simulink model "HumanoidModel_ResidualRL"  (R2025b)
settings: Solver=daessc  StartTime=0.0  StopTime=11  RelTol=1e-3  AbsTol=1e-3
PreLoadFcn:
  | addpath(fullfile('ImportedURDFSupport','Geometries'));
  | addpath(fullfile('ImportedURDFSupport','Data'));
undefined symbols (not defined in the file): kd_ankle_vy, kd_ankle_wx, kd_hip_sag_vx, kd_hip_sag_wy, kd_hip_vy, kd_hip_vz, kd_hip_wx, kp_ankle_qx, kp_ankle_y, kp_hip_dz, kp_hip_qx, kp_hip_sag_qy, kp_hip_sag_x, kp_hip_y, params, residualRLActionPenaltyWeight, residualRLActionRatePenaltyWeight, residualRLAliveReward, residualRLChannelMap, residualRLEnabled, residualRLLeftFootLoadMap, residualRLManualAction, residualRLNominalFootLoad_N, residualRLObservationInverseScales, residualRLRewardStateWeights, residualRLRightFootLoadMap, residualRLSampleTime_s, residualRLTerminalPenalty, residualRLTorqueLimit_Nm, residualRLUseAgent, robustnessForceDuration_s, robustnessForceStart_s, robustnessForceVector_N, Rx_ref, u_ankle_pitch, u_hip_frontal, u_hip_sagittal, u_knee, u_shoulder_frontal, X, Y, y_ref, Z
libraries: sm_lib x155, nesl_utility x96, simulink_extras x18, simulink x5, robotmaniplib x1, rllib x1
(part 1 of 6)
CloseFcn:
  | rmpath(fullfile('ImportedURDFSupport','Geometries'));
  | rmpath(fullfile('ImportedURDFSupport','Data'));
  | clear simlogImportedURDF
settings Model: Creator=The MathWorks, Inc.  LastModifiedBy=EE_LAPTOP_1137
settings SolverCC: AllowMultiTaskInputOutput=on  AlgebraicLoopSolver=TrustRegion
settings OptimizationCC: EnhancedBackFolding=on  OptimizeBlockOrder=speed  DifferentSizesBufferReuse=on  OptimizationCustomize=off
settings DebuggingCC: UnconnectedInputMsg=warning  UnconnectedOutputMsg=warning  UnconnectedLineMsg=warning  SubsystemReferenceDiagnosticForUnitTest=warning  ArithmeticOperatorsInVariantConditions=warning
settings ModelReferenceCC: EnableRefExpFcnMdlSchedulingChecks=on
settings SFSimCC: SimUseLocalCustomCode=off  CustomCodeUndefinedFunction=UseInterfaceOnly
settings RTWCC: RTWUseLocalCustomCode=off  GPUComputeCapability=3.5  DLArmComputeVersion=19.05
settings SimscapeCC: SimscapeLogType=all  SimscapeLogSimulationStatistics=on  SimscapeLogName=simlogImportedURDF  SimscapeLogLimitData=off  SimscapeLogDataHistory=10000.0
settings ExplorerConfigSet: InternalSimMechanicsExplorerSettings="<ExplorerConfiguration><canonicalview>default</canonicalview><AnimationSetting><BasePlaybackSpeed>1.0</BasePlaybackSpeed><PlaybackSpeedFactor>1.0</PlaybackSpeedFactor></AnimationSetting><TilePanel><TileInfo><Tiles Columns=\"1\" Count=\"1\" Rows=\"1\"><Column Weight=\"1\"/><Row Weight=\"1\"/><Tile Height=\"1\" Width=\"1\" X=\"0\" Y=\"0\"/></Tiles></TileInfo><SceneInfo><SceneViewer><BGColor><R>0.60000002384185791</R><G>0.60000002384185791</G><B>0.60000002384185791</B></BGColor><Camera><DoPerspective>off</DoPerspective><Position><X>0.568799300004328878</X><Y>-0.586338342699650017</Y><Z>0.364238790575057481</Z></Position><Center><X>-0.00855096918529698463</X><Y>-0.00898807351002428589</Y><Z>-0.213111478614568334</Z></Center><Up><X>-0.408248290463863073</X><Y>0.408248290463863073</Y><Z>0.816496580927726145</Z></Up><ViewLimDist>1</ViewLimDist><YLim>0.2580841216444969</YLim><XLim>0.471925251007080049</XLim></Camera></SceneViewer></SceneInfo></TilePanel><MechEditorPanel><Cameras/><GfxPanelCameraMap/><VideoCreator><PlaybackSpeedRatio>1.0</PlaybackSpeedRatio><FrameRate>30</FrameRate><VideoFormat>Motion JPEG AVI</VideoFormat><FrameSize>auto</FrameSize></VideoCreator></MechEditorPanel></ExplorerConfiguration>"

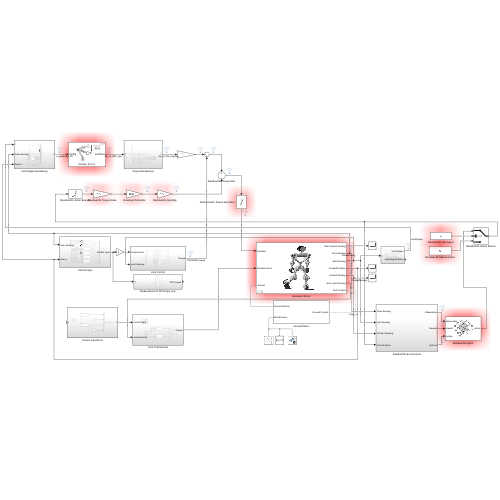
[thumbnail: Simulink's stored preview of the top-level diagram]
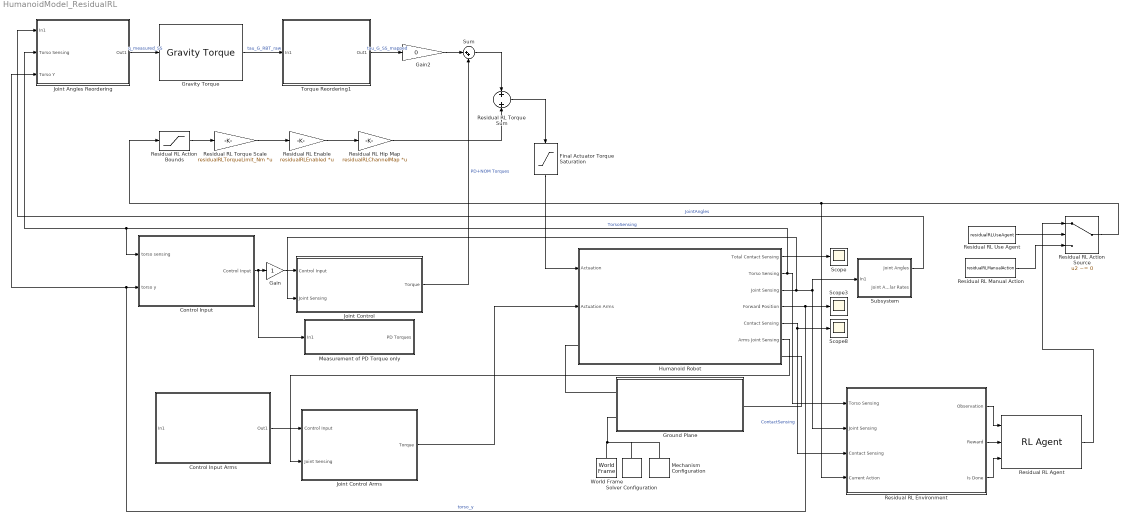
== system HumanoidModel_ResidualRL ==
  Control Input : Subsystem
  Control Input Arms : Subsystem
  Final Actuator Torque Saturation : Saturate  UpperLimit=params.torqueLimits.legActuator  LowerLimit=-params.torqueLimits.legActuator
  Gain : Gain
  Gain2 : Gain  Gain=0
  Gravity Torque : robotmaniplib/Gravity Torque  RigidBodyTree=robotFull  SimulateUsing=Interpreted execution
  Ground Plane : Subsystem
  Humanoid Robot : Subsystem  AncestorBlock=sm_humanoid_walker_lib/Humanoid Robot  mask{contactRadius=params.contact.contactRadius, contactStiffness=params.contact.stiffness, contactDamping=params.contact.damping, contactTWidth=params.contact.transitionWidth, contactStaticFriction=params.contact.staticFriction, contactDynamicFriction=params.contact.dynamicFriction, contactCriticalVelocity=params.contact.criticalVelocity, footDensity=params.materialProperties.lowerBodyDensity, lowerLegDensity=params.materialProperties.lowerBodyDensity, upperLegDensity=params.materialProperties.lowerBodyDensity, hipDensity=params.materialProperties.lowerBodyDensity, trunkDensity=params.materialProperties.upperBodyDensity, shoulderDensity=params.materialProperties.upperBodyDensity, upperArmDensity=params.materialProperties.upperBodyDensity, lowerArmDensity=params.materialProperties.upperBodyDensity, handDensity=params.materialProperties.upperBodyDensity, headDensity=params.materialProperties.upperBodyDensity, hipUpperLimit=params.jointLimits.hipFrontalUpperLimit, hipLowerLimit=params.jointLimits.hipFrontalLowerLimit, kneeUpperLimit=params.jointLimits.kneeUpperLimit, kneeLowerLimit=params.jointLimits.kneeLowerLimit, ankleUpperLimit=params.jointLimits.ankleUpperLimit, ankleLowerLimit=params.jointLimits.ankleLowerLimit, shoulderFrontalUpperLimit=params.jointLimits.shoulderFrontalUpperLimit, shoulderFrontalLowerLimit=params.jointLimits.shoulderFrontalLowerLimit, shoulderSagittalUpperLimit=params.jointLimits.shoulderSagittalUpperLimit, shoulderSagittalLowerLimit=params.jointLimits.shoulderSagittalLowerLimit}
      mask prompts: contactRadius "Contact Sphere Radius (m)"; contactStiffness "Contact Stiffness (N/m)"; contactDamping "Contact Damping (Ns/m)"; contactTWidth "Contact Tranisiton Region Width (m)"; contactStaticFriction "Contact Static Friction"; contactDynamicFriction "Contact Dynamic Friction"; contactCriticalVelocity "Contact Critical Velocity (m/s)"; footDensity "Foot Density (kg/m^3)"; lowerLegDensity "Lower Leg Density (kg/m^3)"; upperLegDensity "Upper Leg Density (kg/m^3)"; hipDensity "Hip Density (kg/m^3)"; trunkDensity "Trunk Density (kg/m^3)"; shoulderDensity "Shoulder Density (kg/m^3)"; upperArmDensity "Upper Arm Density (kg/m^3)"; lowerArmDensity "Lower Arm Density (kg/m^3)"; handDensity "Hand Density (kg/m^3)"; headDensity "Neck / Head Density (kg/m^3)"; hipUpperLimit "Hip Frontal Upper Limit (deg)"; hipLowerLimit "Hip Frontal Lower Limit (deg)"; kneeUpperLimit "Knee Upper Limit (deg)"; kneeLowerLimit "Knee Lower Limit (deg)"; ankleUpperLimit "Ankle Upper Limit (deg)"; ankleLowerLimit "Ankle Lower Limit (deg)"; shoulderFrontalUpperLimit "Shoulder Frontal Upper Limit (deg)"; shoulderFrontalLowerLimit "Shoulder Frontal Lower Limit (deg)"; shoulderSagittalUpperLimit "Shoulder Sagittal Upper Limit (deg)"; shoulderSagittalLowerLimit "Shoulder Sagittal Lower Limit (deg)"
      mask DialogControl Container4 Prompt: Contact Parameters
      mask DialogControl Container9 Prompt: Material Properties
      mask DialogControl Container12 Prompt: Joint Parameters
      mask Display: image('sm_humanoid_robot.PNG'); % Use "Edit Image" on toolstrip to change.
  Joint Angles Reordering : Subsystem
  Joint Control : Subsystem
  Joint Control Arms : Subsystem
  Measurement of PD Torque only : Subsystem
  Mechanism Configuration : sm_lib/Utilities/Mechanism Configuration  UniformGravity=Constant  GravityVector=[0 0 -9.80665]  GravityVectorUnits=m/s^2  LinearizationDelta=0.001  JointModeTransitionNonlinearIterations=2
  Residual RL Action Bounds : Saturate  UpperLimit=1  LowerLimit=-1
  Residual RL Action Source : Switch  Criteria=u2 ~= 0  SaturateOnIntegerOverflow=off  InputSameDT=off
  Residual RL Agent : rllib/RL Agent  Agent=agentObj  ExternalActionAsInput=off  ProvideLastAction=off  ProvideCumRwd=off  TreatAsDirectFeedthrough=on  UseStrictObservationDataTypes=off
  Residual RL Enable : Gain  Gain=residualRLEnabled  Multiplication=Matrix(K*u)
  Residual RL Environment : Subsystem
  Residual RL Hip Map : Gain  Gain=residualRLChannelMap  Multiplication=Matrix(K*u)
  Residual RL Manual Action : Constant  Value=residualRLManualAction
  Residual RL Torque Scale : Gain  Gain=residualRLTorqueLimit_Nm  Multiplication=Matrix(K*u)
  Residual RL Torque Sum : Sum
  Residual RL Use Agent : Constant  Value=residualRLUseAgent
  Scope : Scope
      settings: ActiveDisplayYMinimum=-1  ActiveDisplayYMaximum=1
  Scope3 : Scope
      settings: ActiveDisplayYMinimum=-1.5819424686950212  ActiveDisplayYMaximum=0.4729027116406388  DataLoggingVariableName=ScopeData3
  Scope8 : Scope
      settings: ActiveDisplayYMinimum=-1  ActiveDisplayYMaximum=1  DataLoggingVariableName=ScopeData9
  Solver Configuration : nesl_utility/Solver Configuration  PhysicalDomain=network_engine_domain  SubClassName=solver  LeftPortType=input  RightPortType=generic  Tones=[]  Harmonics=[]  SimulateNoise=off  Profile=off  UseLocalSampling=off  EnableSwitchedLinearOptims=on  FrequencyDomain=off  UseCCode=off  RelTol=0.001  AbsTol=1e-06  MinStep=1e-09  ToWorkspace=off  RevertToSquareIcSolve=off  NumHomotopyIterations=100  PhasorMode=off  PhasorModeNumHarmonics=1  ConsistencySolver=NEWTON_FTOL  IndexReductionMethod=DerivativeReplacement  DoDC=off  ResidualTolerance=1e-09  ConsistencyTolSource=GLOBAL  ConsistencyAbsTol=0.001  ConsistencyRelTol=0.001  ConsistencyTolFactor=0.001  UseLocalSolver=off  LocalSolverChoice=NE_BACKWARD_EULER_ADVANCER  ResolveIndetEquations=on  FunctionEvalNumThread=1  LocalSolverSampleTime=0.001  DoFixedCost=off  MaxNonlinIter=3  MaxModeIter=2  ComputeImpulses=off  ImpulseIterations=2  LinearAlgebra=auto  LinearAlgebraNumThread=0  EquationFormulation=NE_TIME_EF  DelaysMemoryBudget=1024  AutomaticFiltering=on  FilteringTimeConstant=0.001  PartitionStorageMethod=AS_NEEDED  PartitionMemoryBudget=1024  PartitionMethod=ROBUST  MultibodyUseLocalSolver=off  MultibodyLocalSolverChoice=ODE1  MultibodyLocalSolverSampleTime=0.001
  Subsystem : Subsystem
  Sum : Sum  Inputs=|++
  Torque Reordering1 : Subsystem
  World Frame : sm_lib/Frames and Transforms/World Frame
  wires:
  Humanoid Robot/1(Total Contact Sensing) -> Scope/1
  Humanoid Robot/4(Forward Position) -> Joint Angles Reordering/3(Torso Y), Control Input/2(torso y), Scope3/1  "torso_y"
  Humanoid Robot/2(Torso Sensing) -> Joint Angles Reordering/2(Torso Sensing), Control Input/1(torso sensing), Residual RL Environment/1(Torso Sensing)  "TorsoSensing"
  Humanoid Robot/3(Joint Sensing) -> Residual RL Environment/2(Joint Sensing), Subsystem/1(In1), Joint Control/2(Joint Sensing)
  Control Input/1(Control Input) -> Measurement of PD Torque only/1(In1), Gain/1
  Subsystem/1(Joint Angles) -> Joint Angles Reordering/1(In1)  "JointAngles"
  Gain/1 -> Joint Control/1(Control Input)
  Joint Control/1(Torque) -> Sum/2  "PD+NOM Torques"
  Humanoid Robot/5(Contact Sensing) -> Scope8/1, Residual RL Environment/3(Contact Sensing)  "ContactSensing"
  Gain2/1 -> Sum/1
  Joint Angles Reordering/1(Out1) -> Gravity Torque/1  "q_measured_SS"
  Gravity Torque/1 -> Torque Reordering1/1(In1)  "tau_G_RBT_raw"
  Torque Reordering1/1(Out1) -> Gain2/1  "tau_G_SS_mapped"
  Joint Control Arms/1(Torque) -> Humanoid Robot/2(Actuation Arms)
  Control Input Arms/1(Out1) -> Joint Control Arms/1(Control Input)
  Humanoid Robot/6(Arms Joint Sensing) -> Joint Control Arms/2(Joint Sensing)
  Final Actuator Torque Saturation/1 -> Humanoid Robot/1(Actuation)
  Residual RL Action Bounds/1 -> Residual RL Torque Scale/1
  Residual RL Torque Scale/1 -> Residual RL Enable/1
  Residual RL Enable/1 -> Residual RL Hip Map/1
  Sum/1 -> Residual RL Torque Sum/1
  Residual RL Hip Map/1 -> Residual RL Torque Sum/2
  Residual RL Torque Sum/1 -> Final Actuator Torque Saturation/1
  Residual RL Agent/1 -> Residual RL Action Source/1
  Residual RL Use Agent/1 -> Residual RL Action Source/2
  Residual RL Manual Action/1 -> Residual RL Action Source/3
  Residual RL Action Source/1 -> Residual RL Action Bounds/1, Residual RL Environment/4(Current Action)
  Residual RL Environment/1(Observation) -> Residual RL Agent/1
  Residual RL Environment/2(Reward) -> Residual RL Agent/2
  Residual RL Environment/3(Is Done) -> Residual RL Agent/3
  connections:
  Ground Plane/LConn1 -- Humanoid Robot/LConn1
  Ground Plane/LConn2 -- World Frame/RConn1 -- Solver Configuration/RConn1 -- Mechanism Configuration/RConn1
  Humanoid Robot/RConn1 -- Ground Plane/RConn1

== system HumanoidModel_ResidualRL/Control Input ==
  torso sensing : Inport
  torso y : Inport  Port=2
  Bus Selector : BusSelector  OutputSignals=signal1.qx,signal2.wx,signal2.vy,signal2.dz,signal2.vz,signal1.qy,signal2.wy,signal2.x,signal2.vx
  Constant1 : Constant  Value=u_knee
  Constant{5..6,10..11} (4 alike) : Constant  Value=0
  Constant7 : Constant  Value=u_knee
  Left ankle feedback : Subsystem
  Left hip feedback : Subsystem
  Left hip sagittal feedback : Subsystem
  Mux : Mux  Inputs=12
  PD+NOM U : Scope
      settings: ActiveDisplayYMinimum=-15.774140704017688  ActiveDisplayYMaximum=20.952690020044734  DataLoggingVariableName=ScopeData4
  Right ankle feedback : Subsystem
  Right hip feedback : Subsystem
  Right hip sagittal feedback : Subsystem
  Control Input : Outport
  wires:
  Right hip feedback/1(Out1) -> Mux/1  "Right Hip Frontal"
  Mux/1 -> PD+NOM U/1, Control Input/1
  Constant1/1 -> Mux/2  "Right Knee"
  Right ankle feedback/1(Out1) -> Mux/3  "Right Ankle Pitch"
  Right hip sagittal feedback/1(Out1) -> Mux/4  "Right Hip Sagittal"
  Constant5/1 -> Mux/5  "Right Hip Transverse"
  Constant6/1 -> Mux/6  "Right Ankle Roll"
  Constant7/1 -> Mux/8  "Left Knee"
  Left ankle feedback/1(Out1) -> Mux/9  "Left Ankle Pitch"
  Constant11/1 -> Mux/12  "Left Ankle Roll"
  Constant10/1 -> Mux/11  "Left Hip Transverse"
  Left hip sagittal feedback/1(Out1) -> Mux/10  "Left Hip Sagittal"
  torso sensing/1 -> Bus Selector/1
  Bus Selector/1 -> Left hip feedback/1(qx), Left ankle feedback/1(qx), Right ankle feedback/1(qx), Right hip feedback/1(qx)  "<qx>"
  Bus Selector/2 -> Left ankle feedback/2(wx), Left hip feedback/2(wx), Right ankle feedback/2(wx), Right hip feedback/2(wx)  "<wx>"
  Bus Selector/3 -> Right hip feedback/3(vy), Left hip feedback/3(vy), Left ankle feedback/3(vy), Right ankle feedback/3(vy)  "<vy>"
  torso y/1 -> Left hip feedback/4(y), Left ankle feedback/4(y), Right ankle feedback/4(y), Right hip feedback/4(y)
  Left hip feedback/1(Out1) -> Mux/7  "Left Hip Frontal"
  Bus Selector/4 -> Left hip feedback/5(dz), Right hip feedback/5(dz)  "<dz>"
  Bus Selector/5 -> Left hip feedback/6(vz), Right hip feedback/6(vz)  "<vz>"
  Bus Selector/6 -> Left hip sagittal feedback/1(qy), Right hip sagittal feedback/1(qy)  "<qy>"
  Bus Selector/7 -> Left hip sagittal feedback/2(wy), Right hip sagittal feedback/2(wy)  "<wy>"
  Bus Selector/8 -> Left hip sagittal feedback/3(x), Right hip sagittal feedback/3(x)  "<x>"
  Bus Selector/9 -> Left hip sagittal feedback/4(vx), Right hip sagittal feedback/4(vx)  "<vx>"

== system HumanoidModel_ResidualRL/Control Input Arms ==
  In1 : Inport
  Constant1 : Constant  Value=u_shoulder_frontal
  Constant2 : Constant  Value=u_shoulder_frontal
  Constant3 : Constant  Value=0
  Constant5 : Constant  Value=0
  Mux : Mux
  Out1 : Outport
  wires:
  Mux/1 -> Out1/1
  Constant1/1 -> Mux/1  "Right Shoulder Frontal"
  Constant2/1 -> Mux/3  "Left Shoulder Frontal"
  Constant5/1 -> Mux/2  "Right Shoulder Sagittal"
  Constant3/1 -> Mux/4  "Left Shoulder Sagittal"

== system HumanoidModel_ResidualRL/Ground Plane ==
  Ground : sm_lib/Body Elements/Brick Solid  BrickDimensions=[params.display.planeWidth params.display.planeLength params.display.planeHeight]  BrickDimensionsUnits=m  ExportEntireGeometry=on  InertiaType=CalculateFromGeometry  BasedOnType=Density  Density=1000  DensityUnits=kg/m^3  Mass=1  MassUnits=kg  CenterOfMass=[0 0 0]  CenterOfMassUnits=m  MomentsOfInertia=[1 1 1]  MomentsOfInertiaUnits=kg*m^2  ProductsOfInertia=[0 0 0]  ProductsOfInertiaUnits=kg*m^2  GraphicType=FromGeometry  MarkerShape=Sphere  MarkerSize=10  GraphicVisPropType=SimpleVisualProperties  GraphicDiffuseColor=params.display.floorColour  GraphicOpacity=0.3  GraphicSpecularColor=[0.5 0.5 0.5 1.0]  GraphicAmbientColor=[0.15 0.15 0.15 1.0]  GraphicEmissiveColor=[0.0 0.0 0.0 1.0]  GraphicShininess=75  DoExposeReferenceFrame=on  SerializedFrames=<Frames><Frame><Id>Frame1</Id><Value><Name>GS</Name><Origin><Source>GeometricFeature</Source><FeatureName>+z surface</FeatureName></Origin><PrimaryAxis><DefinedDirection>+Z</DefinedDirection><Source>ReferenceFrame</Source><SourceDirection>+Z</SourceDirection><FeatureName></FeatureName></PrimaryAxis><SecondaryAxis><DefinedDirection>+X</DefinedDirection><Source>ReferenceFrame</Source><SourceDirection>+X</SourceDirection><FeatureName></FeatureName></SecondaryAxis></Value></Frame></Frames>
  Rigid Transform : sm_lib/Frames and Transforms/Rigid Transform  RotationMethod=None  FollAlignAxisA=+X  BaseAlignAxisA=+Y  FollAlignAxisB=+Y  BaseAlignAxisB=+Z  RotationStandardAxis=+Z  RotationAngle=0.0  RotationAngleUnits=deg  RotationArbitraryAxis=[0 0 1]  RotationSequenceAxes=FollowerAxes  RotationSequence=XYX  RotationSequenceAngles=[0 0 0]  RotationSequenceAnglesUnits=deg  RotationMatrix=[1 0 0; 0 1 0; 0 0 1]  Quaternion=[1 0 0 0]  TranslationMethod=StandardAxis  TranslationCartesianOffset=[0 0 0]  TranslationCartesianOffsetUnits=m  TranslationStandardAxis=+Y  TranslationStandardOffset=0.5-(params.display.planeLength/2)  TranslationStandardOffsetUnits=m  TranslationROffset=0  TranslationROffsetUnits=m  TranslationThetaOffset=0  TranslationThetaOffsetUnits=deg  TranslationZOffset=0  TranslationZOffsetUnits=m
  Ground Surface : PMIOPort  Side=Left
  Ground Contact : PMIOPort  Port=2  Side=Right
  World Frame : PMIOPort  Port=3  Side=Left
  connections:
  Ground/LConn1 -- Rigid Transform/LConn1
  Ground/LConn2 -- Ground Contact/RConn1
  Ground/RConn1 -- World Frame/RConn1
  Rigid Transform/RConn1 -- Ground Surface/RConn1

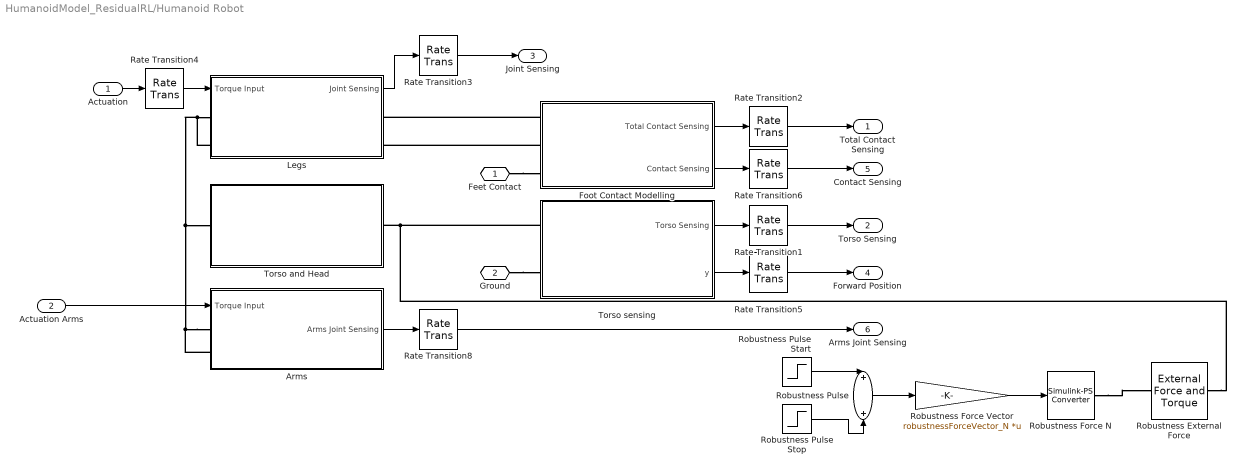
== system HumanoidModel_ResidualRL/Humanoid Robot ==
  Actuation : Inport
  Actuation Arms : Inport  Port=2
  Arms : Subsystem
      mask Display: image('sm_humanoid_arms.PNG'); % Use "Edit Image" on toolstrip to change.
  Foot Contact Modelling : Subsystem
  Legs : Subsystem
      mask Display: image('sm_humanoid_legs.PNG'); % Use "Edit Image" on toolstrip to change.
  Rate Transition{1..6,8} (7 alike) : RateTransition  OutPortSampleTime=params.simulation.Ts
  Robustness External Force : sm_lib/Forces and Torques/External Force and Torque  EnableForceX=off  EnableForceY=off  EnableForceZ=off  EnableForce=on  ForceResolutionFrame=World  EnableTorqueX=off  EnableTorqueY=off  EnableTorqueZ=off  EnableTorque=off  TorqueResolutionFrame=AttachedFrame
  Robustness Force N : nesl_utility/Simulink-PS Converter  PhysicalDomain=network_engine_domain  SubClassName=ps_input  LeftPortType=input  RightPortType=output  PseudoPeriodic=off  Frequencies=[]  NoiseDistribution=none  NoiseParameters=[]  Unit=N  AffineConversion=off  FilteringAndDerivatives=provide  SimscapeFilterOrder=1  InputFilterTimeConstant=0.001  UdotUserProvided=0
  Robustness Force Vector : Gain  Gain=robustnessForceVector_N  Multiplication=Matrix(K*u)
  Robustness Pulse : Sum
  Robustness Pulse Start : Step  Time=robustnessForceStart_s  SampleTime=0
  Robustness Pulse Stop : Step  Time=robustnessForceStart_s + robustnessForceDuration_s  After=-1  SampleTime=0
  Torso and Head : Subsystem
      mask Display: image('sm_humanoid_torso.PNG'); % Use "Edit Image" on toolstrip to change.
  Torso sensing : Subsystem
  Feet Contact : PMIOPort  Side=Right
  " Ground" : PMIOPort  Port=2  Side=Left
  Total Contact Sensing : Outport
  Torso Sensing : Outport  Port=2
  Joint Sensing : Outport  Port=3
  Forward Position : Outport  Port=4
  Contact Sensing : Outport  Port=5
  Arms Joint Sensing : Outport  Port=6
  wires:
  Torso sensing/2(y) -> Rate Transition5/1
  Rate Transition5/1 -> Forward Position/1
  Rate Transition4/1 -> Legs/1(Torque Input)
  Rate Transition3/1 -> Joint Sensing/1
  Rate Transition1/1 -> Torso Sensing/1
  Rate Transition2/1 -> Total Contact Sensing/1
  Torso sensing/1(Torso Sensing) -> Rate Transition1/1
  Actuation/1 -> Rate Transition4/1
  Legs/1(Joint Sensing) -> Rate Transition3/1
  Foot Contact Modelling/1(Total Contact Sensing) -> Rate Transition2/1
  Rate Transition6/1 -> Contact Sensing/1
  Foot Contact Modelling/2(Contact Sensing) -> Rate Transition6/1
  Actuation Arms/1 -> Arms/1(Torque Input)
  Arms/1(Arms Joint Sensing) -> Rate Transition8/1
  Rate Transition8/1 -> Arms Joint Sensing/1
  Robustness Pulse Start/1 -> Robustness Pulse/1
  Robustness Pulse Stop/1 -> Robustness Pulse/2
  Robustness Pulse/1 -> Robustness Force Vector/1
  Robustness Force Vector/1 -> Robustness Force N/1
  connections:
  " Ground"/RConn1 -- Torso sensing/LConn2
  Foot Contact Modelling/LConn2 -- Legs/RConn2
  Foot Contact Modelling/LConn1 -- Legs/RConn1
  Feet Contact/RConn1 -- Foot Contact Modelling/LConn3
  Torso sensing/LConn1 -- Torso and Head/RConn1 -- Robustness External Force/RConn1
  Arms/LConn1 -- Torso and Head/LConn1 -- Legs/LConn1 -- Legs/LConn2 -- Arms/LConn2
  Robustness Force N/RConn1 -- Robustness External Force/LConn1

== system HumanoidModel_ResidualRL/Joint Angles Reordering ==
  In1 : Inport
  Torso Sensing : Inport  Port=2
  Torso Y : Inport  Port=3
  Bus Creator3 : BusCreator  Inputs=22
  Constant : Constant  Value=0
  Demux : Demux  Outputs=12
  Floating Base Selector : BusSelector  OutputSignals=signal2.x,signal2.dz,signal1.qx,signal1.qy,signal1.qz
  Out1 : Outport
  wires:
  In1/1 -> Demux/1
  Bus Creator3/1 -> Out1/1
  Constant/1 -> Bus Creator3/10, Bus Creator3/9, Bus Creator3/8, Bus Creator3/7
  Demux/1 -> Bus Creator3/12  "right_hip_frontal"
  Demux/2 -> Bus Creator3/18  "left_hip_frontal"
  Demux/3 -> Bus Creator3/11  "right_hip_transverse"
  Demux/4 -> Bus Creator3/17  "left_hip_transverse"
  Demux/5 -> Bus Creator3/13  "right_hip_sagittal"
  Demux/6 -> Bus Creator3/19  "left_hip_sagittal"
  Demux/7 -> Bus Creator3/16  "right_ankle_pitch"
  Demux/8 -> Bus Creator3/22  "left_ankle_pitch"
  Demux/9 -> Bus Creator3/15  "right_ankle_roll"
  Demux/10 -> Bus Creator3/21  "left_ankle_roll"
  Demux/11 -> Bus Creator3/14  "right_knee"
  Demux/12 -> Bus Creator3/20  "left_knee"
  Torso Sensing/1 -> Floating Base Selector/1
  Floating Base Selector/1 -> Bus Creator3/1  "<x>"
  Torso Y/1 -> Bus Creator3/2
  Floating Base Selector/2 -> Bus Creator3/3  "<dz>"
  Floating Base Selector/3 -> Bus Creator3/4  "<qx>"
  Floating Base Selector/4 -> Bus Creator3/5  "<qy>"
  Floating Base Selector/5 -> Bus Creator3/6  "<qz>"

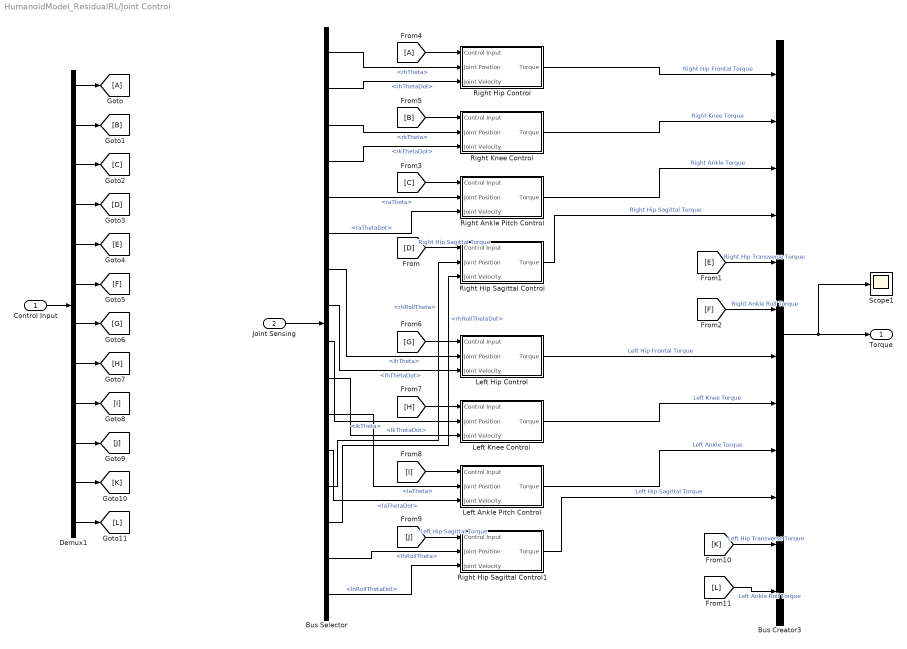
== system HumanoidModel_ResidualRL/Joint Control ==
  Control Input : Inport
  Joint Sensing : Inport  Port=2
  Bus Creator3 : BusCreator  Inputs=12
  Bus Selector : BusSelector  OutputSignals=signal1.signal1.rhTheta,signal1.signal1.rhThetaDot,signal1.signal2.rkTheta,signal1.signal2.rkThetaDot,signal1.signal3.raTheta,signal1.signal3.raThetaDot,signal2.signal1.lhTheta,signal2.signal1.lhThetaDot,signal2.signal2.lkTheta,signal2.signal2.lkThetaDot,signal2.signal3.laTheta,signal2.signal3.laThetaDot,signal1.signal4.rhRollTheta,signal1.signal4.rhRollThetaDot,signal2.signal4.lhRollTheta,signal2.signal4.lhRollThetaDot
  Demux1 : Demux  Outputs=12
  From4 : From
  Goto : Goto
  Left Ankle Pitch Control : Subsystem  AncestorBlock=sm_humanoid_walker_lib/Joint Controller  mask{jointStiffness=params.controller.ankleStiffness, jointDamping=params.controller.ankleDamping, jointUpperLimit=params.jointLimits.ankleUpperLimit, jointLowerLimit=params.jointLimits.ankleLowerLimit, jointTorqueLimit=params.torqueLimits.ankle}
      mask prompts: jointStiffness "Joint Control Stiffness (N*m/rad)"; jointDamping "Joint Control Damping (N*m*s/rad)"; jointUpperLimit "Joint Upper Limit (deg)"; jointLowerLimit "Joint Lower Limt (deg)"; jointTorqueLimit "Joint Absolute Torque Limit (N*m)"
      mask DialogControl DescTextVar Prompt: Stiffness based joint controller.
  Left Hip Control : Subsystem  AncestorBlock=sm_humanoid_walker_lib/Joint Controller  mask{jointStiffness=params.controller.hipFrontalStiffness, jointDamping=params.controller.hipFrontalDamping, jointUpperLimit=params.jointLimits.hipFrontalUpperLimit, jointLowerLimit=params.jointLimits.hipFrontalLowerLimit, jointTorqueLimit=params.torqueLimits.hipFrontal}
      mask prompts: jointStiffness "Joint Control Stiffness (N*m/rad)"; jointDamping "Joint Control Damping (N*m*s/rad)"; jointUpperLimit "Joint Upper Limit (deg)"; jointLowerLimit "Joint Lower Limt (deg)"; jointTorqueLimit "Joint Absolute Torque Limit (N*m)"
      mask DialogControl DescTextVar Prompt: Stiffness based joint controller.
  Left Knee Control : Subsystem  AncestorBlock=sm_humanoid_walker_lib/Joint Controller  mask{jointStiffness=params.controller.kneeStiffness, jointDamping=params.controller.kneeDamping, jointUpperLimit=params.jointLimits.kneeUpperLimit, jointLowerLimit=params.jointLimits.kneeLowerLimit, jointTorqueLimit=params.torqueLimits.knee}
      mask prompts: jointStiffness "Joint Control Stiffness (N*m/rad)"; jointDamping "Joint Control Damping (N*m*s/rad)"; jointUpperLimit "Joint Upper Limit (deg)"; jointLowerLimit "Joint Lower Limt (deg)"; jointTorqueLimit "Joint Absolute Torque Limit (N*m)"
      mask DialogControl DescTextVar Prompt: Stiffness based joint controller.
  Right Ankle Pitch Control : Subsystem  AncestorBlock=sm_humanoid_walker_lib/Joint Controller  mask{jointStiffness=params.controller.ankleStiffness, jointDamping=params.controller.ankleDamping, jointUpperLimit=params.jointLimits.ankleUpperLimit, jointLowerLimit=params.jointLimits.ankleLowerLimit, jointTorqueLimit=params.torqueLimits.ankle}
      mask prompts: jointStiffness "Joint Control Stiffness (N*m/rad)"; jointDamping "Joint Control Damping (N*m*s/rad)"; jointUpperLimit "Joint Upper Limit (deg)"; jointLowerLimit "Joint Lower Limt (deg)"; jointTorqueLimit "Joint Absolute Torque Limit (N*m)"
      mask DialogControl DescTextVar Prompt: Stiffness based joint controller.
  Right Hip Control : Subsystem  AncestorBlock=sm_humanoid_walker_lib/Joint Controller  mask{jointStiffness=params.controller.hipFrontalStiffness, jointDamping=params.controller.hipFrontalDamping, jointUpperLimit=params.jointLimits.hipFrontalUpperLimit, jointLowerLimit=params.jointLimits.hipFrontalLowerLimit, jointTorqueLimit=params.torqueLimits.hipFrontal}
      mask prompts: jointStiffness "Joint Control Stiffness (N*m/rad)"; jointDamping "Joint Control Damping (N*m*s/rad)"; jointUpperLimit "Joint Upper Limit (deg)"; jointLowerLimit "Joint Lower Limt (deg)"; jointTorqueLimit "Joint Absolute Torque Limit (N*m)"
      mask DialogControl DescTextVar Prompt: Stiffness based joint controller.
  Right Hip Sagittal Control : Subsystem  AncestorBlock=sm_humanoid_walker_lib/Joint Controller  mask{jointStiffness=params.controller.hipSagittalStiffness, jointDamping=params.controller.hipSagittalDamping, jointUpperLimit=params.jointLimits.hipSagittalUpperLimit, jointLowerLimit=params.jointLimits.hipSagittalLowerLimit, jointTorqueLimit=params.torqueLimits.hipSagittal}
      mask prompts: jointStiffness "Joint Control Stiffness (N*m/rad)"; jointDamping "Joint Control Damping (N*m*s/rad)"; jointUpperLimit "Joint Upper Limit (deg)"; jointLowerLimit "Joint Lower Limt (deg)"; jointTorqueLimit "Joint Absolute Torque Limit (N*m)"
      mask DialogControl DescTextVar Prompt: Stiffness based joint controller.
  Right Hip Sagittal Control1 : Subsystem  AncestorBlock=sm_humanoid_walker_lib/Joint Controller  mask{jointStiffness=params.controller.hipSagittalStiffness, jointDamping=params.controller.hipSagittalDamping, jointUpperLimit=params.jointLimits.hipSagittalUpperLimit, jointLowerLimit=params.jointLimits.hipSagittalLowerLimit, jointTorqueLimit=params.torqueLimits.hipSagittal}
      mask prompts: jointStiffness "Joint Control Stiffness (N*m/rad)"; jointDamping "Joint Control Damping (N*m*s/rad)"; jointUpperLimit "Joint Upper Limit (deg)"; jointLowerLimit "Joint Lower Limt (deg)"; jointTorqueLimit "Joint Absolute Torque Limit (N*m)"
      mask DialogControl DescTextVar Prompt: Stiffness based joint controller.
  Right Knee Control : Subsystem  AncestorBlock=sm_humanoid_walker_lib/Joint Controller  mask{jointStiffness=params.controller.kneeStiffness, jointDamping=params.controller.kneeDamping, jointUpperLimit=params.jointLimits.kneeUpperLimit, jointLowerLimit=params.jointLimits.kneeLowerLimit, jointTorqueLimit=params.torqueLimits.knee}
      mask prompts: jointStiffness "Joint Control Stiffness (N*m/rad)"; jointDamping "Joint Control Damping (N*m*s/rad)"; jointUpperLimit "Joint Upper Limit (deg)"; jointLowerLimit "Joint Lower Limt (deg)"; jointTorqueLimit "Joint Absolute Torque Limit (N*m)"
      mask DialogControl DescTextVar Prompt: Stiffness based joint controller.
  Scope1 : Scope
      settings: ActiveDisplayYMinimum=-18.809813505018703  ActiveDisplayYMaximum=29.661981385621988  DataLoggingVariableName=ScopeData8
  Torque : Outport
  wires:
  Right Hip Control/1(Torque) -> Bus Creator3/1  "Right Hip Frontal Torque"
  [B] -> Right Knee Control/1(Control Input)
  Bus Creator3/1 -> Scope1/1, Torque/1
  Demux1/3 -> [C]
  [I] -> Left Ankle Pitch Control/1(Control Input)
  Bus Selector/10 -> Left Knee Control/3(Joint Velocity)  "<lkThetaDot>"
  Demux1/1 -> Goto/1
  Right Ankle Pitch Control/1(Torque) -> Bus Creator3/3  "Right Ankle Torque"
  Bus Selector/3 -> Right Knee Control/2(Joint Position)  "<rkTheta>"
  Bus Selector/6 -> Right Ankle Pitch Control/3(Joint Velocity)  "<raThetaDot>"
  Bus Selector/11 -> Left Ankle Pitch Control/2(Joint Position)  "<laTheta>"
  Bus Selector/12 -> Left Ankle Pitch Control/3(Joint Velocity)  "<laThetaDot>"
  [C] -> Right Ankle Pitch Control/1(Control Input)
  Right Knee Control/1(Torque) -> Bus Creator3/2  "Right Knee Torque"
  Bus Selector/4 -> Right Knee Control/3(Joint Velocity)  "<rkThetaDot>"
  Bus Selector/1 -> Right Hip Control/2(Joint Position)  "<rhTheta>"
  [H] -> Left Knee Control/1(Control Input)
  Bus Selector/9 -> Left Knee Control/2(Joint Position)  "<lkTheta>"
  Control Input/1 -> Demux1/1
  Joint Sensing/1 -> Bus Selector/1
  From4/1 -> Right Hip Control/1(Control Input)
  Bus Selector/7 -> Left Hip Control/2(Joint Position)  "<lhTheta>"
  Bus Selector/2 -> Right Hip Control/3(Joint Velocity)  "<rhThetaDot>"
  Demux1/5 -> [E]
  Bus Selector/8 -> Left Hip Control/3(Joint Velocity)  "<lhThetaDot>"
  Demux1/2 -> [B]
  Bus Selector/5 -> Right Ankle Pitch Control/2(Joint Position)  "<raTheta>"
  [G] -> Left Hip Control/1(Control Input)
  Demux1/4 -> [D]
  Demux1/6 -> [F]
  Demux1/7 -> [G]
  Demux1/8 -> [H]
  Demux1/9 -> [I]
  Demux1/10 -> [J]
  Demux1/11 -> [K]
  Demux1/12 -> [L]
  Left Ankle Pitch Control/1(Torque) -> Bus Creator3/9  "Left Ankle Torque"
  Left Knee Control/1(Torque) -> Bus Creator3/8  "Left Knee Torque"
  Left Hip Control/1(Torque) -> Bus Creator3/7  "Left Hip Frontal Torque"
  [L] -> Bus Creator3/12  "Left Ankle Roll Torque"
  [K] -> Bus Creator3/11  "Left Hip Transverse Torque"
  [F] -> Bus Creator3/6  "Right Ankle Roll Torque"
  [E] -> Bus Creator3/5  "Right Hip Transverse Torque"
  [D] -> Right Hip Sagittal Control/1(Control Input)  "Right Hip Sagittal Torque"
  Right Hip Sagittal Control/1(Torque) -> Bus Creator3/4  "Right Hip Sagittal Torque"
  Bus Selector/13 -> Right Hip Sagittal Control/2(Joint Position)  "<rhRollTheta>"
  Bus Selector/14 -> Right Hip Sagittal Control/3(Joint Velocity)  "<rhRollThetaDot>"
  Right Hip Sagittal Control1/1(Torque) -> Bus Creator3/10  "Left Hip Sagittal Torque"
  [J] -> Right Hip Sagittal Control1/1(Control Input)  "Left Hip Sagittal Torque"
  Bus Selector/15 -> Right Hip Sagittal Control1/2(Joint Position)  "<lhRollTheta>"
  Bus Selector/16 -> Right Hip Sagittal Control1/3(Joint Velocity)  "<lhRollThetaDot>"

== system HumanoidModel_ResidualRL/Joint Control Arms ==
  Control Input : Inport
  Joint Sensing : Inport  Port=2
  Bus Selector : BusSelector  OutputSignals=signal1.signal1.rsfTheta,signal2.signal1.lsfThetaDot,signal2.signal1.lsfTheta,signal1.signal1.rsfThetaDot
  Demux1 : Demux
  From : From
  Goto : Goto
  Left Shoulder Frontal Control : Subsystem  AncestorBlock=sm_humanoid_walker_lib/Joint Controller  mask{jointStiffness=params.controller.hipFrontalStiffness, jointDamping=params.controller.hipFrontalDamping, jointUpperLimit=params.jointLimits.hipFrontalUpperLimit, jointLowerLimit=params.jointLimits.hipFrontalLowerLimit, jointTorqueLimit=params.torqueLimits.hipFrontal}
      mask prompts: jointStiffness "Joint Control Stiffness (N*m/rad)"; jointDamping "Joint Control Damping (N*m*s/rad)"; jointUpperLimit "Joint Upper Limit (deg)"; jointLowerLimit "Joint Lower Limt (deg)"; jointTorqueLimit "Joint Absolute Torque Limit (N*m)"
      mask DialogControl DescTextVar Prompt: Stiffness based joint controller.
  Mux : Mux
  PD_Torques_Arms : Scope
      settings: ActiveDisplayYMinimum=-8.9552249091287219  ActiveDisplayYMaximum=7.6438983308339683  DataLoggingVariableName=ScopeData2
  Right Shoulder Frontal Control : Subsystem  AncestorBlock=sm_humanoid_walker_lib/Joint Controller  mask{jointStiffness=params.controller.hipFrontalStiffness, jointDamping=params.controller.hipFrontalDamping, jointUpperLimit=params.jointLimits.hipFrontalUpperLimit, jointLowerLimit=params.jointLimits.hipFrontalLowerLimit, jointTorqueLimit=params.torqueLimits.hipFrontal}
      mask prompts: jointStiffness "Joint Control Stiffness (N*m/rad)"; jointDamping "Joint Control Damping (N*m*s/rad)"; jointUpperLimit "Joint Upper Limit (deg)"; jointLowerLimit "Joint Lower Limt (deg)"; jointTorqueLimit "Joint Absolute Torque Limit (N*m)"
      mask DialogControl DescTextVar Prompt: Stiffness based joint controller.
  Torque : Outport
  wires:
  Right Shoulder Frontal Control/1(Torque) -> Mux/1  "Right Shoulder Frontal Torque"
  Joint Sensing/1 -> Bus Selector/1
  Control Input/1 -> Demux1/1
  Demux1/1 -> Goto/1
  Demux1/2 -> [B]
  Demux1/3 -> [C]
  Demux1/4 -> [D]
  From/1 -> Right Shoulder Frontal Control/1(Control Input)
  Left Shoulder Frontal Control/1(Torque) -> Mux/3  "Left Shoulder Frontal Torque"
  [C] -> Left Shoulder Frontal Control/1(Control Input)
  [B] -> Mux/2
  [D] -> Mux/4
  Bus Selector/1 -> Right Shoulder Frontal Control/2(Joint Position)  "<rsfTheta>"
  Bus Selector/2 -> Right Shoulder Frontal Control/3(Joint Velocity)  "<lsfThetaDot>"
  Bus Selector/3 -> Left Shoulder Frontal Control/2(Joint Position)  "<lsfTheta>"
  Bus Selector/4 -> Left Shoulder Frontal Control/3(Joint Velocity)  "<rsfThetaDot>"
  Mux/1 -> PD_Torques_Arms/1, Torque/1

== system HumanoidModel_ResidualRL/Measurement of PD Torque only ==
  In1 : Inport
  Demux : Demux  Outputs=12
  Left Ankle Pitch Control : Subsystem  AncestorBlock=sm_humanoid_walker_lib/Joint Controller  mask{jointStiffness=params.controller.ankleStiffness, jointDamping=params.controller.ankleDamping, jointUpperLimit=params.jointLimits.ankleUpperLimit, jointLowerLimit=params.jointLimits.ankleLowerLimit, jointTorqueLimit=params.torqueLimits.ankle}
      mask prompts: jointStiffness "Joint Control Stiffness (N*m/rad)"; jointDamping "Joint Control Damping (N*m*s/rad)"; jointUpperLimit "Joint Upper Limit (deg)"; jointLowerLimit "Joint Lower Limt (deg)"; jointTorqueLimit "Joint Absolute Torque Limit (N*m)"
      mask DialogControl DescTextVar Prompt: Stiffness based joint controller.
  Left Hip Control : Subsystem  AncestorBlock=sm_humanoid_walker_lib/Joint Controller  mask{jointStiffness=params.controller.hipFrontalStiffness, jointDamping=params.controller.hipFrontalDamping, jointUpperLimit=params.jointLimits.hipFrontalUpperLimit, jointLowerLimit=params.jointLimits.hipFrontalLowerLimit, jointTorqueLimit=params.torqueLimits.hipFrontal}
      mask prompts: jointStiffness "Joint Control Stiffness (N*m/rad)"; jointDamping "Joint Control Damping (N*m*s/rad)"; jointUpperLimit "Joint Upper Limit (deg)"; jointLowerLimit "Joint Lower Limt (deg)"; jointTorqueLimit "Joint Absolute Torque Limit (N*m)"
      mask DialogControl DescTextVar Prompt: Stiffness based joint controller.
  Left Knee Control : Subsystem  AncestorBlock=sm_humanoid_walker_lib/Joint Controller  mask{jointStiffness=params.controller.kneeStiffness, jointDamping=params.controller.kneeDamping, jointUpperLimit=params.jointLimits.kneeUpperLimit, jointLowerLimit=params.jointLimits.kneeLowerLimit, jointTorqueLimit=params.torqueLimits.knee}
      mask prompts: jointStiffness "Joint Control Stiffness (N*m/rad)"; jointDamping "Joint Control Damping (N*m*s/rad)"; jointUpperLimit "Joint Upper Limit (deg)"; jointLowerLimit "Joint Lower Limt (deg)"; jointTorqueLimit "Joint Absolute Torque Limit (N*m)"
      mask DialogControl DescTextVar Prompt: Stiffness based joint controller.
  Mux : Mux  Inputs=12
  Nominal u : Subsystem
  Right Ankle Pitch Control : Subsystem  AncestorBlock=sm_humanoid_walker_lib/Joint Controller  mask{jointStiffness=params.controller.ankleStiffness, jointDamping=params.controller.ankleDamping, jointUpperLimit=params.jointLimits.ankleUpperLimit, jointLowerLimit=params.jointLimits.ankleLowerLimit, jointTorqueLimit=params.torqueLimits.ankle}
      mask prompts: jointStiffness "Joint Control Stiffness (N*m/rad)"; jointDamping "Joint Control Damping (N*m*s/rad)"; jointUpperLimit "Joint Upper Limit (deg)"; jointLowerLimit "Joint Lower Limt (deg)"; jointTorqueLimit "Joint Absolute Torque Limit (N*m)"
      mask DialogControl DescTextVar Prompt: Stiffness based joint controller.
  Right Hip Control : Subsystem  AncestorBlock=sm_humanoid_walker_lib/Joint Controller  mask{jointStiffness=params.controller.hipFrontalStiffness, jointDamping=params.controller.hipFrontalDamping, jointUpperLimit=params.jointLimits.hipFrontalUpperLimit, jointLowerLimit=params.jointLimits.hipFrontalLowerLimit, jointTorqueLimit=params.torqueLimits.hipFrontal}
      mask prompts: jointStiffness "Joint Control Stiffness (N*m/rad)"; jointDamping "Joint Control Damping (N*m*s/rad)"; jointUpperLimit "Joint Upper Limit (deg)"; jointLowerLimit "Joint Lower Limt (deg)"; jointTorqueLimit "Joint Absolute Torque Limit (N*m)"
      mask DialogControl DescTextVar Prompt: Stiffness based joint controller.
  Right Hip Sagittal Control : Subsystem  AncestorBlock=sm_humanoid_walker_lib/Joint Controller  mask{jointStiffness=params.controller.hipSagittalStiffness, jointDamping=params.controller.hipSagittalDamping, jointUpperLimit=params.jointLimits.hipSagittalUpperLimit, jointLowerLimit=params.jointLimits.hipSagittalLowerLimit, jointTorqueLimit=params.torqueLimits.hipSagittal}
      mask prompts: jointStiffness "Joint Control Stiffness (N*m/rad)"; jointDamping "Joint Control Damping (N*m*s/rad)"; jointUpperLimit "Joint Upper Limit (deg)"; jointLowerLimit "Joint Lower Limt (deg)"; jointTorqueLimit "Joint Absolute Torque Limit (N*m)"
      mask DialogControl DescTextVar Prompt: Stiffness based joint controller.
  Right Hip Sagittal Control1 : Subsystem  AncestorBlock=sm_humanoid_walker_lib/Joint Controller  mask{jointStiffness=params.controller.hipSagittalStiffness, jointDamping=params.controller.hipSagittalDamping, jointUpperLimit=params.jointLimits.hipSagittalUpperLimit, jointLowerLimit=params.jointLimits.hipSagittalLowerLimit, jointTorqueLimit=params.torqueLimits.hipSagittal}
      mask prompts: jointStiffness "Joint Control Stiffness (N*m/rad)"; jointDamping "Joint Control Damping (N*m*s/rad)"; jointUpperLimit "Joint Upper Limit (deg)"; jointLowerLimit "Joint Lower Limt (deg)"; jointTorqueLimit "Joint Absolute Torque Limit (N*m)"
      mask DialogControl DescTextVar Prompt: Stiffness based joint controller.
  Right Knee Control : Subsystem  AncestorBlock=sm_humanoid_walker_lib/Joint Controller  mask{jointStiffness=params.controller.kneeStiffness, jointDamping=params.controller.kneeDamping, jointUpperLimit=params.jointLimits.kneeUpperLimit, jointLowerLimit=params.jointLimits.kneeLowerLimit, jointTorqueLimit=params.torqueLimits.knee}
      mask prompts: jointStiffness "Joint Control Stiffness (N*m/rad)"; jointDamping "Joint Control Damping (N*m*s/rad)"; jointUpperLimit "Joint Upper Limit (deg)"; jointLowerLimit "Joint Lower Limt (deg)"; jointTorqueLimit "Joint Absolute Torque Limit (N*m)"
      mask DialogControl DescTextVar Prompt: Stiffness based joint controller.
  Scope : Scope
      settings: ActiveDisplayYMinimum=-15.024947891967964  ActiveDisplayYMaximum=17.12220363288316  DataLoggingVariableName=ScopeData6
  Sum : Sum  Inputs=|-+
  PD Torques : Outport
  wires:
  Nominal u/1(Out1) -> Sum/1
  In1/1 -> Sum/2
  Sum/1 -> Demux/1
  Demux/1 -> Right Hip Control/1(Control Input)
  Demux/2 -> Right Knee Control/1(Control Input)
  Demux/3 -> Right Ankle Pitch Control/1(Control Input)
  Demux/4 -> Right Hip Sagittal Control/1(Control Input)
  Demux/7 -> Left Hip Control/1(Control Input)
  Demux/8 -> Left Knee Control/1(Control Input)
  Demux/9 -> Left Ankle Pitch Control/1(Control Input)
  Right Hip Control/1(Torque) -> Mux/1  "Right Hip Frontal Torque"
  Right Knee Control/1(Torque) -> Mux/2  "Right Knee Torque"
  Right Ankle Pitch Control/1(Torque) -> Mux/3  "Right Ankle Torque"
  Right Hip Sagittal Control/1(Torque) -> Mux/4  "Right Hip Sagittal Torque"
  Left Knee Control/1(Torque) -> Mux/8  "Left Knee Torque"
  Left Ankle Pitch Control/1(Torque) -> Mux/9  "Left Ankle Torque"
  Right Hip Sagittal Control1/1(Torque) -> Mux/10  "Left Hip Sagittal Torque"
  Demux/10 -> Right Hip Sagittal Control1/1(Control Input)
  Demux/5 -> Mux/5  "Right Hip Transverse Torque"
  Demux/6 -> Mux/6  "Right Ankle Roll Torque"
  Left Hip Control/1(Torque) -> Mux/7  "Left Hip Frontal Torque"
  Demux/11 -> Mux/11  "Left Hip Transverse Torque"
  Demux/12 -> Mux/12  "Left Ankle Roll Torque"
  Mux/1 -> Scope/1, PD Torques/1  "Pure PD Torques"

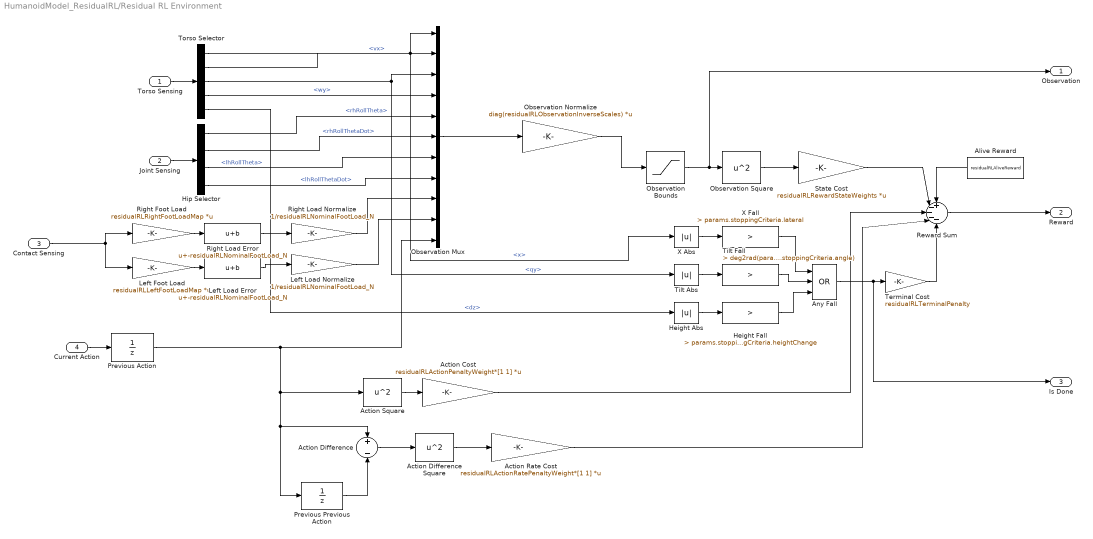
== system HumanoidModel_ResidualRL/Residual RL Environment ==
  Torso Sensing : Inport
  Joint Sensing : Inport  Port=2
  Contact Sensing : Inport  Port=3
  Current Action : Inport  Port=4
  Action Cost : Gain  Gain=residualRLActionPenaltyWeight*[1 1]  Multiplication=Matrix(K*u)
  Action Difference : Sum  Inputs=+-
  Action Difference Square : Math  Operator=square
  Action Rate Cost : Gain  Gain=residualRLActionRatePenaltyWeight*[1 1]  Multiplication=Matrix(K*u)
  Action Square : Math  Operator=square
  Alive Reward : Constant  Value=residualRLAliveReward
  Any Fall : Logic  Operator=OR  Inputs=3  AllPortsSameDT=off  OutDataTypeStr=boolean
  Height Abs : Abs  SaturateOnIntegerOverflow=off
  Height Fall : simulink/Logic and Bit Operations/Compare To Constant  relop=>  const=params.stoppingCriteria.heightChange  OutDataTypeStr=boolean
  Hip Selector : BusSelector  OutputSignals=signal1.signal4.rhRollTheta,signal1.signal4.rhRollThetaDot,signal2.signal4.lhRollTheta,signal2.signal4.lhRollThetaDot
  Left Foot Load : Gain  Gain=residualRLLeftFootLoadMap  Multiplication=Matrix(K*u)
  Left Load Error : Bias  Bias=-residualRLNominalFootLoad_N  SaturateOnIntegerOverflow=off
  Left Load Normalize : Gain  Gain=1/residualRLNominalFootLoad_N
  Observation Bounds : Saturate  UpperLimit=5  LowerLimit=-5
  Observation Mux : Mux  Inputs=11
  Observation Normalize : Gain  Gain=diag(residualRLObservationInverseScales)  Multiplication=Matrix(K*u)
  Observation Square : Math  Operator=square
  Previous Action : UnitDelay  InitialCondition=zeros(2,1)  SampleTime=residualRLSampleTime_s  HasFrameUpgradeWarning=on
  Previous Previous Action : UnitDelay  InitialCondition=zeros(2,1)  SampleTime=residualRLSampleTime_s  HasFrameUpgradeWarning=on
  Reward Sum : Sum  Inputs=+----
  Right Foot Load : Gain  Gain=residualRLRightFootLoadMap  Multiplication=Matrix(K*u)
  Right Load Error : Bias  Bias=-residualRLNominalFootLoad_N  SaturateOnIntegerOverflow=off
  Right Load Normalize : Gain  Gain=1/residualRLNominalFootLoad_N
  State Cost : Gain  Gain=residualRLRewardStateWeights  Multiplication=Matrix(K*u)
  Terminal Cost : Gain  Gain=residualRLTerminalPenalty
  Tilt Abs : Abs  SaturateOnIntegerOverflow=off
  Tilt Fall : simulink/Logic and Bit Operations/Compare To Constant  relop=>  const=deg2rad(params.stoppingCriteria.angle)  OutDataTypeStr=boolean
  Torso Selector : BusSelector  OutputSignals=signal2.x,signal2.vx,signal1.qy,signal2.wy,signal2.dz
  X Abs : Abs  SaturateOnIntegerOverflow=off
  X Fall : simulink/Logic and Bit Operations/Compare To Constant  relop=>  const=params.stoppingCriteria.lateral  OutDataTypeStr=boolean
  Observation : Outport
  Reward : Outport  Port=2
  Is Done : Outport  Port=3
  wires:
  X Abs/1 -> X Fall/1
  Tilt Abs/1 -> Tilt Fall/1
  Height Abs/1 -> Height Fall/1
  Torso Sensing/1 -> Torso Selector/1
  Joint Sensing/1 -> Hip Selector/1
  Contact Sensing/1 -> Left Foot Load/1, Right Foot Load/1
  Right Foot Load/1 -> Right Load Error/1
  Right Load Error/1 -> Right Load Normalize/1
  Left Foot Load/1 -> Left Load Error/1
  Left Load Error/1 -> Left Load Normalize/1
  Current Action/1 -> Previous Action/1
  Previous Action/1 -> Previous Previous Action/1, Action Difference/1, Action Square/1, Observation Mux/11
  Torso Selector/1 -> Observation Mux/1, X Abs/1  "<x>"
  Torso Selector/2 -> Observation Mux/2  "<vx>"
  Torso Selector/3 -> Tilt Abs/1, Observation Mux/3  "<qy>"
  Torso Selector/4 -> Observation Mux/4  "<wy>"
  Hip Selector/1 -> Observation Mux/5  "<rhRollTheta>"
  Hip Selector/2 -> Observation Mux/6  "<rhRollThetaDot>"
  Hip Selector/3 -> Observation Mux/7  "<lhRollTheta>"
  Hip Selector/4 -> Observation Mux/8  "<lhRollThetaDot>"
  Right Load Normalize/1 -> Observation Mux/9
  Left Load Normalize/1 -> Observation Mux/10
  Observation Mux/1 -> Observation Normalize/1
  Observation Normalize/1 -> Observation Bounds/1
  Observation Bounds/1 -> Observation Square/1, Observation/1
  Observation Square/1 -> State Cost/1
  Action Square/1 -> Action Cost/1
  Previous Previous Action/1 -> Action Difference/2
  Action Difference/1 -> Action Difference Square/1
  Action Difference Square/1 -> Action Rate Cost/1
  Torso Selector/5 -> Height Abs/1  "<dz>"
  X Fall/1 -> Any Fall/1
  Tilt Fall/1 -> Any Fall/2
  Height Fall/1 -> Any Fall/3
  Any Fall/1 -> Is Done/1, Terminal Cost/1
  Alive Reward/1 -> Reward Sum/1
  State Cost/1 -> Reward Sum/2
  Action Cost/1 -> Reward Sum/3
  Action Rate Cost/1 -> Reward Sum/4
  Terminal Cost/1 -> Reward Sum/5
  Reward Sum/1 -> Reward/1

== system HumanoidModel_ResidualRL/Subsystem ==
  In1 : Inport
  Bus Creator2 : BusCreator  Inputs=12
  Bus Creator3 : BusCreator  Inputs=12
  Bus Selector : BusSelector  OutputSignals=signal1.signal1.rhTheta,signal2.signal5.lhYawThetaDot,signal2.signal5.lhYawTheta,signal2.signal4.lhRollThetaDot,signal2.signal4.lhRollTheta,signal2.signal3.laRollThetaDot,signal2.signal3.laRollTheta,signal2.signal3.laThetaDot,signal2.signal3.laTheta,signal2.signal2.lkThetaDot,signal2.signal2.lkTheta,signal2.signal1.lhThetaDot,signal2.signal1.lhTheta,signal1.signal5.rhYawThetaDot,signal1.signal5.rhYawTheta,signal1.signal4.rhRollThetaDot,signal1.signal4.rhRollTheta,signal1.signal3.raRollThetaDot,signal1.signal3.raRollTheta,signal1.signal3.raThetaDot,signal1.signal3.raTheta,signal1.signal2.rkThetaDot,signal1.signal2.rkTheta,signal1.signal1.rhThetaDot
  Scope4 : Scope
      settings: ActiveDisplayYMinimum=-0.34043292838947647  ActiveDisplayYMaximum=0.26375673911123687  DataLoggingVariableName=ScopeData10
  Joint Angles : Outport
  Joint Angular Rates : Outport  Port=2
  wires:
  In1/1 -> Bus Selector/1
  Bus Selector/23 -> Bus Creator2/11  "<rkTheta>"
  Bus Selector/22 -> Bus Creator3/11  "<rkThetaDot>"
  Bus Selector/21 -> Bus Creator2/7  "<raTheta>"
  Bus Selector/20 -> Bus Creator3/7  "<raThetaDot>"
  Bus Selector/19 -> Bus Creator2/9  "<raRollTheta>"
  Bus Selector/18 -> Bus Creator3/9  "<raRollThetaDot>"
  Bus Selector/17 -> Bus Creator2/5  "<rhRollTheta>"
  Bus Selector/16 -> Bus Creator3/5  "<rhRollThetaDot>"
  Bus Selector/15 -> Bus Creator2/3  "<rhYawTheta>"
  Bus Selector/14 -> Bus Creator3/3  "<rhYawThetaDot>"
  Bus Selector/13 -> Bus Creator2/2  "<lhTheta>"
  Bus Selector/12 -> Bus Creator3/2  "<lhThetaDot>"
  Bus Selector/11 -> Bus Creator2/12  "<lkTheta>"
  Bus Selector/10 -> Bus Creator3/12  "<lkThetaDot>"
  Bus Selector/9 -> Bus Creator2/8  "<laTheta>"
  Bus Selector/8 -> Bus Creator3/8  "<laThetaDot>"
  Bus Selector/7 -> Bus Creator2/10  "<laRollTheta>"
  Bus Selector/6 -> Bus Creator3/10  "<laRollThetaDot>"
  Bus Selector/5 -> Bus Creator2/6  "<lhRollTheta>"
  Bus Selector/4 -> Bus Creator3/6  "<lhRollThetaDot>"
  Bus Selector/3 -> Bus Creator2/4  "<lhYawTheta>"
  Bus Selector/2 -> Bus Creator3/4  "<lhYawThetaDot>"
  Bus Selector/1 -> Bus Creator2/1  "<rhTheta>"
  Bus Selector/24 -> Bus Creator3/1  "<rhThetaDot>"
  Bus Creator3/1 -> Joint Angular Rates/1
  Bus Creator2/1 -> Scope4/1, Joint Angles/1
